simulink model "LookupTableND_test_1D_nearest"  (R2017b)
settings: Solver=FixedStepDiscrete  StartTime=0.0  StopTime=10.0  FixedStep=0.200000  RelTol=1e-3  EnableMultiTasking=on
settings Model: Creator=hbourbou  LastModifiedBy=hbourbou
settings DataIOCC: LimitDataPoints=on  SaveFormat=StructureWithTime
settings OptimizationCC: LifeSpan=inf
settings DebuggingCC: SFUnexpectedBacktrackingDiag=warning  SFNoUnconditionalDefaultTransitionDiag=warning  SFExecutionAtInitializationDiag=none
settings HardwareCC: ProdBitPerSizeT=32  ProdBitPerPtrDiffT=32  ProdWordSize=32  ProdHWDeviceType=Specified
settings ModelReferenceCC: PropagateSignalLabelsOutOfModel=off
settings CodeAppCC: StateflowObjectComments=on
settings GRTTargetCC: TargetLangStandard=C89/C90 (ANSI)
settings ConfigComp: CovMetricSettings=dw  CovHtmlReporting=on  CovSaveCumulativeToWorkspaceVar=on  CovSaveSingleToWorkspaceVar=on  CovExternalEMLEnable=off

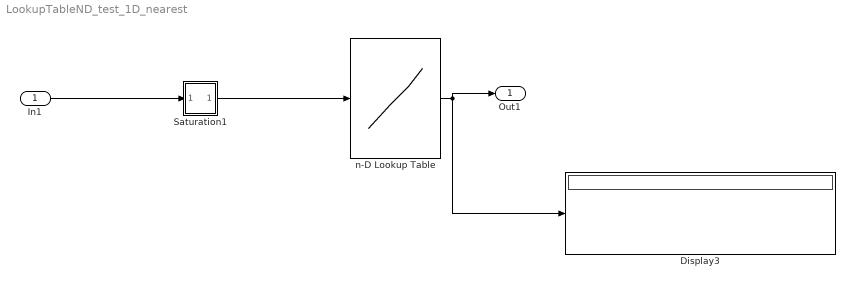
== system LookupTableND_test_1D_nearest ==
  In1 : Inport
  Display3 : Display
  Saturation1 : Subsystem  TreatAsAtomicUnit=on
      settings: MinAlgLoopOccurrences=on
  n-D Lookup Table : Lookup_n-D  NumberOfTableDimensions=1  BreakpointsForDimension1="[0 1.5 2.2  3.1]"  BreakpointsForDimension2=[4 5 6]  BreakpointsForDimension3=[5 6]  UseOneInputPortForAllInputData=on  Table=[10 110 120 230]  InterpMethod=Nearest  InternalRulePriority=Speed  RndMeth=Simplest  InputSameDT=on
  Out1 : Outport
  wires:
  n-D Lookup Table/1 -> Out1/1, Display3/1
  Saturation1/1(Out) -> n-D Lookup Table/1
  In1/1 -> Saturation1/1(In)

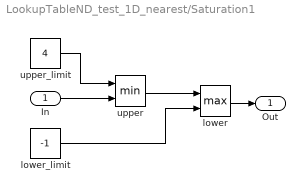
== system LookupTableND_test_1D_nearest/Saturation1 ==
  In : Inport
  lower : MinMax  Function=max  Inputs=2
  lower_limit : Constant  Value=-1  SampleTime=-1
  upper : MinMax  Inputs=2
  upper_limit : Constant  Value=4  SampleTime=-1
  Out : Outport
  wires:
  lower/1 -> Out/1
  In/1 -> upper/2
  lower_limit/1 -> lower/2
  upper/1 -> lower/1
  upper_limit/1 -> upper/1
